simulink model "Kugle_sys7_block"  (R2018b)
settings: Solver=VariableStepAuto  StartTime=0.0  StopTime=10.0  RelTol=1e-3
settings Model: Creator=martinandersen  LastModifiedBy=martinandersen

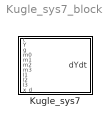
== system Kugle_sys7_block ==
  Kugle_sys7 : MATLAB Function  TreatAsAtomicUnit=on

== matlab function Kugle_sys7_block/Kugle_sys7 ==
  data: t input; dYdt output; Y input; g input; m0 input; m1 input; m2 input; m3 input; l1 input; l2 input; l3 input; x_d input
function dYdt = Kugle_sys7(t,Y,g,m0,m1,m2,m3,l1,l2,l3,x_d)
%#codegen

%    This function was generated by the Symbolic Math Toolbox version 8.2.
%    11-May-2019 12:19:22

t3 = Y(3);
t2 = cos(t3);
t4 = t2.^2;
t5 = m3.^2;
t7 = Y(5);
t6 = cos(t7);
t11 = t3+t7;
t8 = cos(t11);
t9 = m2.^2;
t10 = t6.^2;
t12 = t8.^2;
t13 = Y(1);
t14 = sin(t13);
t15 = Y(2);
t16 = sin(t3);
t17 = t15.^2;
t18 = Y(4);
t19 = t18.^2;
t20 = t3+t13;
t21 = sin(t20);
t22 = sin(t11);
t23 = Y(6);
t24 = t23.^2;
t25 = sin(t7);
t26 = t3+t7+t13;
t27 = sin(t26);
t28 = 1.0./l1;
t29 = t4.*t9.*9.0;
t30 = t4.*t5.*3.6e1;
t31 = t5.*t10.*2.7e1;
t32 = t5.*t12.*2.7e1;
t33 = m2.*m3.*t4.*3.6e1;
t34 = m1.*m3.*t10.*9.0;
t35 = m2.*m3.*t10.*2.7e1;
t36 = m2.*m3.*t12.*9.0;
t37 = t5.*-3.6e1-t9.*1.2e1+t29+t30+t31+t32+t33+t34+t35+t36-m1.*m2.*4.0-m1.*m3.*1.2e1-m2.*m3.*4.8e1-t2.*t5.*t6.*t8.*5.4e1-m2.*m3.*t2.*t6.*t8.*2.7e1;
t38 = 1.0./t37;
t39 = l1.^2;
t40 = l2.^2;
t41 = l3.^2;
dYdt = [t15;t28.*t38.*(g.*t5.*t14.*2.4e1+g.*t9.*t14.*8.0+g.*m1.*m2.*t14.*4.0+g.*m1.*m3.*t14.*1.2e1+g.*m2.*m3.*t14.*3.2e1-g.*t2.*t5.*t21.*2.4e1-g.*t5.*t10.*t14.*1.8e1-g.*t2.*t9.*t21.*6.0-g.*t5.*t8.*t27.*1.8e1+l2.*t5.*t16.*t17.*2.4e1+l2.*t5.*t16.*t19.*2.4e1+l2.*t9.*t16.*t17.*4.0+l2.*t9.*t16.*t19.*4.0+l3.*t5.*t17.*t22.*1.2e1+l3.*t5.*t19.*t22.*1.2e1+l3.*t5.*t22.*t24.*1.2e1-g.*m1.*m3.*t10.*t14.*9.0-g.*m2.*m3.*t2.*t21.*2.4e1-g.*m2.*m3.*t10.*t14.*1.8e1-g.*m2.*m3.*t8.*t27.*6.0+l2.*m2.*m3.*t16.*t17.*2.0e1+l2.*m2.*m3.*t16.*t19.*2.0e1+l3.*m2.*m3.*t17.*t22.*4.0+l3.*m2.*m3.*t19.*t22.*4.0+l3.*m2.*m3.*t22.*t24.*4.0+g.*t2.*t5.*t6.*t27.*1.8e1+g.*t5.*t6.*t8.*t21.*1.8e1+l1.*t2.*t5.*t16.*t17.*2.4e1+l1.*t2.*t9.*t16.*t17.*6.0-l2.*t5.*t10.*t16.*t17.*1.8e1-l2.*t5.*t10.*t16.*t19.*1.8e1-l3.*t2.*t5.*t17.*t25.*1.2e1+l1.*t5.*t8.*t17.*t22.*1.8e1-l3.*t2.*t5.*t19.*t25.*1.2e1+l2.*t5.*t15.*t16.*t18.*4.8e1+l2.*t5.*t8.*t17.*t25.*1.8e1-l3.*t5.*t10.*t17.*t22.*9.0+l2.*t5.*t8.*t19.*t25.*1.8e1-l3.*t2.*t5.*t24.*t25.*1.2e1-l3.*t5.*t10.*t19.*t22.*9.0+l2.*t9.*t15.*t16.*t18.*8.0+l3.*t5.*t15.*t18.*t22.*2.4e1-l3.*t5.*t10.*t22.*t24.*9.0+l3.*t5.*t15.*t22.*t23.*2.4e1+l3.*t5.*t18.*t22.*t23.*2.4e1+l1.*m2.*m3.*t2.*t16.*t17.*2.4e1-l2.*m2.*m3.*t10.*t16.*t17.*9.0-l2.*m2.*m3.*t10.*t16.*t19.*9.0-l3.*m2.*m3.*t2.*t17.*t25.*6.0+l1.*m2.*m3.*t8.*t17.*t22.*6.0-l3.*m2.*m3.*t2.*t19.*t25.*6.0+l2.*m2.*m3.*t15.*t16.*t18.*4.0e1+l2.*m2.*m3.*t8.*t17.*t25.*6.0+l2.*m2.*m3.*t8.*t19.*t25.*6.0-l3.*m2.*m3.*t2.*t24.*t25.*6.0+l3.*m2.*m3.*t15.*t18.*t22.*8.0+l3.*m2.*m3.*t15.*t22.*t23.*8.0+l3.*m2.*m3.*t18.*t22.*t23.*8.0-l1.*t2.*t5.*t6.*t17.*t22.*1.8e1-l1.*t5.*t6.*t8.*t16.*t17.*1.8e1-l2.*t2.*t5.*t6.*t17.*t25.*1.8e1-l2.*t2.*t5.*t6.*t19.*t25.*1.8e1+l3.*t5.*t6.*t8.*t17.*t25.*9.0-l2.*t5.*t10.*t15.*t16.*t18.*3.6e1+l3.*t5.*t6.*t8.*t19.*t25.*9.0-l3.*t2.*t5.*t15.*t18.*t25.*2.4e1+l3.*t5.*t6.*t8.*t24.*t25.*9.0+l2.*t5.*t8.*t15.*t18.*t25.*3.6e1-l3.*t2.*t5.*t15.*t23.*t25.*2.4e1-l3.*t5.*t10.*t15.*t18.*t22.*1.8e1-l3.*t2.*t5.*t18.*t23.*t25.*2.4e1-l3.*t5.*t10.*t15.*t22.*t23.*1.8e1-l3.*t5.*t10.*t18.*t22.*t23.*1.8e1+g.*m2.*m3.*t2.*t6.*t27.*9.0+g.*m2.*m3.*t6.*t8.*t21.*9.0-l1.*m2.*m3.*t2.*t6.*t17.*t22.*9.0-l1.*m2.*m3.*t6.*t8.*t16.*t17.*9.0-l2.*m2.*m3.*t2.*t6.*t17.*t25.*9.0-l2.*m2.*m3.*t2.*t6.*t19.*t25.*9.0-l2.*m2.*m3.*t10.*t15.*t16.*t18.*1.8e1-l3.*m2.*m3.*t2.*t15.*t18.*t25.*1.2e1+l2.*m2.*m3.*t8.*t15.*t18.*t25.*1.2e1-l3.*m2.*m3.*t2.*t15.*t23.*t25.*1.2e1-l3.*m2.*m3.*t2.*t18.*t23.*t25.*1.2e1-l2.*t2.*t5.*t6.*t15.*t18.*t25.*3.6e1+l3.*t5.*t6.*t8.*t15.*t18.*t25.*1.8e1+l3.*t5.*t6.*t8.*t15.*t23.*t25.*1.8e1+l3.*t5.*t6.*t8.*t18.*t23.*t25.*1.8e1-l2.*m2.*m3.*t2.*t6.*t15.*t18.*t25.*1.8e1).*(-3.0./2.0);t18;(t28.*t38.*(g.*l2.*t5.*t14.*2.4e1+g.*l2.*t9.*t14.*8.0-g.*l1.*t5.*t21.*2.4e1-g.*l1.*t9.*t21.*1.2e1+t5.*t16.*t17.*t39.*2.4e1+t5.*t16.*t17.*t40.*2.4e1+t5.*t16.*t19.*t40.*2.4e1+t9.*t16.*t17.*t39.*1.2e1+t9.*t16.*t17.*t40.*4.0+t9.*t16.*t19.*t40.*4.0+g.*l2.*m1.*m2.*t14.*4.0+g.*l2.*m1.*m3.*t14.*1.2e1+g.*l2.*m2.*m3.*t14.*3.2e1-g.*l1.*m1.*m2.*t21.*4.0-g.*l1.*m1.*m3.*t21.*8.0-g.*l1.*m2.*m3.*t21.*3.6e1+g.*l1.*t2.*t5.*t14.*2.4e1+g.*l1.*t2.*t9.*t14.*1.2e1-g.*l2.*t2.*t5.*t21.*2.4e1-g.*l2.*t5.*t10.*t14.*1.8e1-g.*l2.*t2.*t9.*t21.*6.0+g.*l1.*t5.*t6.*t27.*1.8e1+g.*l1.*t5.*t12.*t21.*1.8e1-g.*l2.*t5.*t8.*t27.*1.8e1+l2.*l3.*t5.*t17.*t22.*1.2e1-l1.*l3.*t5.*t17.*t25.*1.2e1+l2.*l3.*t5.*t19.*t22.*1.2e1-l1.*l3.*t5.*t19.*t25.*1.2e1+l2.*l3.*t5.*t22.*t24.*1.2e1-l1.*l3.*t5.*t24.*t25.*1.2e1+m1.*m2.*t16.*t17.*t39.*4.0+m1.*m3.*t16.*t17.*t39.*8.0+m2.*m3.*t16.*t17.*t39.*3.6e1+m2.*m3.*t16.*t17.*t40.*2.0e1+m2.*m3.*t16.*t19.*t40.*2.0e1-t5.*t10.*t16.*t17.*t40.*1.8e1-t5.*t6.*t17.*t22.*t39.*1.8e1-t5.*t12.*t16.*t17.*t39.*1.8e1-t5.*t10.*t16.*t19.*t40.*1.8e1+t5.*t15.*t16.*t18.*t40.*4.8e1+t5.*t8.*t17.*t25.*t40.*1.8e1+t5.*t8.*t19.*t25.*t40.*1.8e1+t9.*t15.*t16.*t18.*t40.*8.0-g.*l1.*t5.*t6.*t8.*t14.*1.8e1+g.*l2.*t2.*t5.*t6.*t27.*1.8e1+g.*l2.*t5.*t6.*t8.*t21.*1.8e1-g.*l1.*t2.*t5.*t8.*t27.*1.8e1+l1.*l2.*t2.*t5.*t16.*t17.*4.8e1+l1.*l2.*t2.*t5.*t16.*t19.*2.4e1+l1.*l2.*t2.*t9.*t16.*t17.*1.2e1+l1.*l2.*t2.*t9.*t16.*t19.*6.0+l1.*l3.*t2.*t5.*t17.*t22.*1.2e1+l1.*l3.*t2.*t5.*t19.*t22.*1.2e1-l2.*l3.*t2.*t5.*t17.*t25.*1.2e1+l1.*l2.*t5.*t8.*t17.*t22.*1.8e1-l1.*l2.*t5.*t6.*t17.*t25.*1.8e1-l2.*l3.*t2.*t5.*t19.*t25.*1.2e1+l1.*l3.*t2.*t5.*t22.*t24.*1.2e1-l1.*l2.*t5.*t6.*t19.*t25.*1.8e1-l2.*l3.*t5.*t10.*t17.*t22.*9.0-l2.*l3.*t2.*t5.*t24.*t25.*1.2e1-l2.*l3.*t5.*t10.*t19.*t22.*9.0+l1.*l3.*t5.*t12.*t17.*t25.*9.0+l1.*l3.*t5.*t12.*t19.*t25.*9.0+l2.*l3.*t5.*t15.*t18.*t22.*2.4e1-l2.*l3.*t5.*t10.*t22.*t24.*9.0-l1.*l3.*t5.*t15.*t18.*t25.*2.4e1+l1.*l3.*t5.*t12.*t24.*t25.*9.0+l2.*l3.*t5.*t15.*t22.*t23.*2.4e1-l1.*l3.*t5.*t15.*t23.*t25.*2.4e1+l2.*l3.*t5.*t18.*t22.*t23.*2.4e1-l1.*l3.*t5.*t18.*t23.*t25.*2.4e1-m1.*m3.*t6.*t17.*t22.*t39.*6.0-m2.*m3.*t10.*t16.*t17.*t40.*9.0-m2.*m3.*t6.*t17.*t22.*t39.*1.8e1-m2.*m3.*t12.*t16.*t17.*t39.*9.0-m2.*m3.*t10.*t16.*t19.*t40.*9.0+m2.*m3.*t15.*t16.*t18.*t40.*4.0e1+m2.*m3.*t8.*t17.*t25.*t40.*6.0+m2.*m3.*t8.*t19.*t25.*t40.*6.0+t2.*t5.*t8.*t17.*t22.*t39.*1.8e1-t2.*t5.*t6.*t17.*t25.*t40.*1.8e1-t2.*t5.*t6.*t19.*t25.*t40.*1.8e1-t5.*t10.*t15.*t16.*t18.*t40.*3.6e1+t5.*t8.*t15.*t18.*t25.*t40.*3.6e1+g.*l1.*m1.*m2.*t2.*t14.*6.0+g.*l1.*m1.*m3.*t2.*t14.*1.2e1+g.*l1.*m2.*m3.*t2.*t14.*3.6e1-g.*l2.*m1.*m3.*t10.*t14.*9.0-g.*l2.*m2.*m3.*t2.*t21.*2.4e1-g.*l2.*m2.*m3.*t10.*t14.*1.8e1+g.*l1.*m1.*m3.*t6.*t27.*6.0+g.*l1.*m2.*m3.*t6.*t27.*1.8e1+g.*l1.*m2.*m3.*t12.*t21.*9.0-g.*l2.*m2.*m3.*t8.*t27.*6.0+l2.*l3.*m2.*m3.*t17.*t22.*4.0-l1.*l3.*m1.*m3.*t17.*t25.*4.0-l1.*l3.*m2.*m3.*t17.*t25.*1.2e1+l2.*l3.*m2.*m3.*t19.*t22.*4.0-l1.*l3.*m1.*m3.*t19.*t25.*4.0-l1.*l3.*m2.*m3.*t19.*t25.*1.2e1+l2.*l3.*m2.*m3.*t22.*t24.*4.0-l1.*l3.*m1.*m3.*t24.*t25.*4.0-l1.*l3.*m2.*m3.*t24.*t25.*1.2e1-g.*l1.*m1.*m3.*t6.*t8.*t14.*9.0-g.*l1.*m2.*m3.*t6.*t8.*t14.*1.8e1+g.*l2.*m2.*m3.*t2.*t6.*t27.*9.0+g.*l2.*m2.*m3.*t6.*t8.*t21.*9.0-g.*l1.*m2.*m3.*t2.*t8.*t27.*9.0+l1.*l2.*m2.*m3.*t2.*t16.*t17.*4.8e1+l1.*l2.*m2.*m3.*t2.*t16.*t19.*2.4e1+l1.*l3.*m2.*m3.*t2.*t17.*t22.*6.0+l1.*l3.*m2.*m3.*t2.*t19.*t22.*6.0-l2.*l3.*m2.*m3.*t2.*t17.*t25.*6.0-l1.*l2.*m1.*m3.*t6.*t17.*t25.*6.0+l1.*l2.*m2.*m3.*t8.*t17.*t22.*6.0-l1.*l2.*m2.*m3.*t6.*t17.*t25.*1.8e1-l2.*l3.*m2.*m3.*t2.*t19.*t25.*6.0-l1.*l2.*m1.*m3.*t6.*t19.*t25.*6.0+l1.*l3.*m2.*m3.*t2.*t22.*t24.*6.0-l1.*l2.*m2.*m3.*t6.*t19.*t25.*1.8e1-l2.*l3.*m2.*m3.*t2.*t24.*t25.*6.0+l2.*l3.*m2.*m3.*t15.*t18.*t22.*8.0-l1.*l3.*m1.*m3.*t15.*t18.*t25.*8.0-l1.*l3.*m2.*m3.*t15.*t18.*t25.*2.4e1+l2.*l3.*m2.*m3.*t15.*t22.*t23.*8.0-l1.*l3.*m1.*m3.*t15.*t23.*t25.*8.0-l1.*l3.*m2.*m3.*t15.*t23.*t25.*2.4e1+l2.*l3.*m2.*m3.*t18.*t22.*t23.*8.0-l1.*l3.*m1.*m3.*t18.*t23.*t25.*8.0-l1.*l3.*m2.*m3.*t18.*t23.*t25.*2.4e1-l1.*l2.*t2.*t5.*t6.*t17.*t22.*1.8e1-l1.*l2.*t5.*t6.*t8.*t16.*t17.*3.6e1-l1.*l2.*t5.*t6.*t8.*t16.*t19.*1.8e1+l1.*l2.*t2.*t5.*t15.*t16.*t18.*4.8e1+l1.*l2.*t2.*t5.*t8.*t17.*t25.*1.8e1+l1.*l2.*t2.*t5.*t8.*t19.*t25.*1.8e1-l1.*l3.*t5.*t6.*t8.*t17.*t22.*9.0+l1.*l2.*t2.*t9.*t15.*t16.*t18.*1.2e1-l1.*l3.*t5.*t6.*t8.*t19.*t22.*9.0+l1.*l3.*t2.*t5.*t15.*t18.*t22.*2.4e1+l2.*l3.*t5.*t6.*t8.*t17.*t25.*9.0+l2.*l3.*t5.*t6.*t8.*t19.*t25.*9.0-l1.*l3.*t5.*t6.*t8.*t22.*t24.*9.0-l2.*l3.*t2.*t5.*t15.*t18.*t25.*2.4e1+l1.*l3.*t2.*t5.*t15.*t22.*t23.*2.4e1-l1.*l2.*t5.*t6.*t15.*t18.*t25.*3.6e1+l2.*l3.*t5.*t6.*t8.*t24.*t25.*9.0+l1.*l3.*t2.*t5.*t18.*t22.*t23.*2.4e1-l2.*l3.*t2.*t5.*t15.*t23.*t25.*2.4e1-l2.*l3.*t5.*t10.*t15.*t18.*t22.*1.8e1-l2.*l3.*t2.*t5.*t18.*t23.*t25.*2.4e1+l1.*l3.*t5.*t12.*t15.*t18.*t25.*1.8e1-l2.*l3.*t5.*t10.*t15.*t22.*t23.*1.8e1-l2.*l3.*t5.*t10.*t18.*t22.*t23.*1.8e1+l1.*l3.*t5.*t12.*t15.*t23.*t25.*1.8e1+l1.*l3.*t5.*t12.*t18.*t23.*t25.*1.8e1+m2.*m3.*t2.*t8.*t17.*t22.*t39.*9.0-m2.*m3.*t2.*t6.*t17.*t25.*t40.*9.0-m2.*m3.*t2.*t6.*t19.*t25.*t40.*9.0-m2.*m3.*t10.*t15.*t16.*t18.*t40.*1.8e1+m2.*m3.*t8.*t15.*t18.*t25.*t40.*1.2e1-t2.*t5.*t6.*t15.*t18.*t25.*t40.*3.6e1-l1.*l2.*m2.*m3.*t2.*t6.*t17.*t22.*9.0-l1.*l2.*m2.*m3.*t6.*t8.*t16.*t17.*1.8e1-l1.*l2.*m2.*m3.*t6.*t8.*t16.*t19.*9.0+l1.*l2.*m2.*m3.*t2.*t15.*t16.*t18.*4.8e1+l1.*l2.*m2.*m3.*t2.*t8.*t17.*t25.*9.0+l1.*l2.*m2.*m3.*t2.*t8.*t19.*t25.*9.0+l1.*l3.*m2.*m3.*t2.*t15.*t18.*t22.*1.2e1-l2.*l3.*m2.*m3.*t2.*t15.*t18.*t25.*1.2e1-l1.*l2.*m1.*m3.*t6.*t15.*t18.*t25.*1.2e1+l1.*l3.*m2.*m3.*t2.*t15.*t22.*t23.*1.2e1-l1.*l2.*m2.*m3.*t6.*t15.*t18.*t25.*3.6e1+l1.*l3.*m2.*m3.*t2.*t18.*t22.*t23.*1.2e1-l2.*l3.*m2.*m3.*t2.*t15.*t23.*t25.*1.2e1-l2.*l3.*m2.*m3.*t2.*t18.*t23.*t25.*1.2e1-l1.*l2.*t5.*t6.*t8.*t15.*t16.*t18.*3.6e1+l1.*l2.*t2.*t5.*t8.*t15.*t18.*t25.*3.6e1-l1.*l3.*t5.*t6.*t8.*t15.*t18.*t22.*1.8e1+l2.*l3.*t5.*t6.*t8.*t15.*t18.*t25.*1.8e1-l1.*l3.*t5.*t6.*t8.*t15.*t22.*t23.*1.8e1-l1.*l3.*t5.*t6.*t8.*t18.*t22.*t23.*1.8e1+l2.*l3.*t5.*t6.*t8.*t15.*t23.*t25.*1.8e1+l2.*l3.*t5.*t6.*t8.*t18.*t23.*t25.*1.8e1-m2.*m3.*t2.*t6.*t15.*t18.*t25.*t40.*1.8e1-l1.*l2.*m2.*m3.*t6.*t8.*t15.*t16.*t18.*1.8e1+l1.*l2.*m2.*m3.*t2.*t8.*t15.*t18.*t25.*1.8e1).*(3.0./2.0))./l2;t23;((g.*l3.*t5.*t21.*2.4e1+g.*l3.*t9.*t21.*1.2e1-g.*l2.*t5.*t27.*3.6e1-g.*l2.*t9.*t27.*1.2e1+t5.*t17.*t25.*t40.*3.6e1+t5.*t17.*t25.*t41.*1.2e1+t5.*t19.*t25.*t40.*3.6e1+t5.*t19.*t25.*t41.*1.2e1+t9.*t17.*t25.*t40.*1.2e1+t9.*t19.*t25.*t40.*1.2e1+t5.*t24.*t25.*t41.*1.2e1+g.*l3.*m1.*m2.*t21.*4.0+g.*l3.*m1.*m3.*t21.*8.0+g.*l3.*m2.*m3.*t21.*3.6e1-g.*l2.*m1.*m2.*t27.*4.0-g.*l2.*m1.*m3.*t27.*1.2e1-g.*l2.*m2.*m3.*t27.*4.8e1-g.*l3.*t2.*t5.*t14.*2.4e1-g.*l3.*t2.*t9.*t14.*1.2e1+g.*l2.*t5.*t8.*t14.*3.6e1+g.*l2.*t8.*t9.*t14.*1.2e1+g.*l2.*t5.*t6.*t21.*3.6e1+g.*l2.*t4.*t5.*t27.*3.6e1+g.*l2.*t6.*t9.*t21.*1.8e1-g.*l3.*t5.*t6.*t27.*1.8e1-g.*l3.*t5.*t12.*t21.*1.8e1+g.*l2.*t4.*t9.*t27.*9.0-l1.*l3.*t5.*t16.*t17.*2.4e1-l1.*l3.*t9.*t16.*t17.*1.2e1+l1.*l2.*t5.*t17.*t22.*3.6e1+l1.*l2.*t9.*t17.*t22.*1.2e1+m1.*m2.*t17.*t25.*t40.*4.0+m1.*m3.*t17.*t25.*t40.*1.2e1+m1.*m2.*t19.*t25.*t40.*4.0+m1.*m3.*t17.*t25.*t41.*4.0+m2.*m3.*t17.*t25.*t40.*4.8e1+m1.*m3.*t19.*t25.*t40.*1.2e1+m2.*m3.*t17.*t25.*t41.*1.2e1+m1.*m3.*t19.*t25.*t41.*4.0+m2.*m3.*t19.*t25.*t40.*4.8e1+m2.*m3.*t19.*t25.*t41.*1.2e1+m1.*m3.*t24.*t25.*t41.*4.0+m2.*m3.*t24.*t25.*t41.*1.2e1+t5.*t8.*t16.*t17.*t40.*3.6e1-t2.*t5.*t17.*t22.*t41.*1.2e1+t5.*t8.*t16.*t19.*t40.*3.6e1-t2.*t5.*t19.*t22.*t41.*1.2e1+t8.*t9.*t16.*t17.*t40.*6.0-t4.*t5.*t17.*t25.*t40.*3.6e1+t8.*t9.*t16.*t19.*t40.*6.0-t4.*t5.*t19.*t25.*t40.*3.6e1-t2.*t5.*t22.*t24.*t41.*1.2e1-t4.*t9.*t17.*t25.*t40.*9.0-t4.*t9.*t19.*t25.*t40.*9.0-t5.*t12.*t17.*t25.*t41.*9.0-t5.*t12.*t19.*t25.*t41.*9.0+t5.*t15.*t18.*t25.*t40.*7.2e1+t5.*t15.*t18.*t25.*t41.*2.4e1-t5.*t12.*t24.*t25.*t41.*9.0+t9.*t15.*t18.*t25.*t40.*2.4e1+t5.*t15.*t23.*t25.*t41.*2.4e1+t5.*t18.*t23.*t25.*t41.*2.4e1-g.*l2.*t2.*t5.*t6.*t14.*3.6e1-g.*l2.*t2.*t6.*t9.*t14.*1.8e1+g.*l3.*t5.*t6.*t8.*t14.*1.8e1-g.*l2.*t2.*t5.*t8.*t21.*3.6e1-g.*l2.*t2.*t8.*t9.*t21.*9.0+g.*l3.*t2.*t5.*t8.*t27.*1.8e1-l2.*l3.*t2.*t5.*t16.*t17.*2.4e1-l1.*l2.*t5.*t6.*t16.*t17.*3.6e1-l2.*l3.*t2.*t5.*t16.*t19.*2.4e1-l2.*l3.*t2.*t9.*t16.*t17.*6.0-l1.*l2.*t4.*t5.*t17.*t22.*3.6e1-l1.*l2.*t6.*t9.*t16.*t17.*1.8e1-l2.*l3.*t2.*t9.*t16.*t19.*6.0+l1.*l3.*t5.*t6.*t17.*t22.*1.8e1+l1.*l3.*t5.*t12.*t16.*t17.*1.8e1-l1.*l2.*t4.*t9.*t17.*t22.*9.0+l2.*l3.*t5.*t8.*t17.*t22.*1.8e1+l2.*l3.*t5.*t6.*t17.*t25.*3.6e1+l2.*l3.*t5.*t8.*t19.*t22.*1.8e1+l2.*l3.*t5.*t6.*t19.*t25.*3.6e1+l2.*l3.*t5.*t8.*t22.*t24.*1.8e1+l2.*l3.*t5.*t6.*t24.*t25.*1.8e1+m2.*m3.*t8.*t16.*t17.*t40.*3.0e1-m2.*m3.*t2.*t17.*t22.*t41.*6.0+m2.*m3.*t8.*t16.*t19.*t40.*3.0e1-m2.*m3.*t2.*t19.*t22.*t41.*6.0-m2.*m3.*t4.*t17.*t25.*t40.*3.6e1-m2.*m3.*t4.*t19.*t25.*t40.*3.6e1-m2.*m3.*t2.*t22.*t24.*t41.*6.0+m1.*m2.*t15.*t18.*t25.*t40.*8.0+m1.*m3.*t15.*t18.*t25.*t40.*2.4e1+m1.*m3.*t15.*t18.*t25.*t41.*8.0+m2.*m3.*t15.*t18.*t25.*t40.*9.6e1+m2.*m3.*t15.*t18.*t25.*t41.*2.4e1+m1.*m3.*t15.*t23.*t25.*t41.*8.0+m2.*m3.*t15.*t23.*t25.*t41.*2.4e1+m1.*m3.*t18.*t23.*t25.*t41.*8.0+m2.*m3.*t18.*t23.*t25.*t41.*2.4e1-t2.*t5.*t6.*t16.*t17.*t40.*3.6e1-t2.*t5.*t6.*t16.*t19.*t40.*3.6e1-t2.*t6.*t9.*t16.*t17.*t40.*9.0-t2.*t6.*t9.*t16.*t19.*t40.*9.0+t5.*t6.*t8.*t17.*t22.*t41.*9.0+t5.*t6.*t8.*t19.*t22.*t41.*9.0+t5.*t8.*t15.*t16.*t18.*t40.*7.2e1-t2.*t5.*t15.*t18.*t22.*t41.*2.4e1+t5.*t6.*t8.*t22.*t24.*t41.*9.0+t8.*t9.*t15.*t16.*t18.*t40.*1.2e1-t4.*t5.*t15.*t18.*t25.*t40.*7.2e1-t2.*t5.*t15.*t22.*t23.*t41.*2.4e1-t2.*t5.*t18.*t22.*t23.*t41.*2.4e1-t4.*t9.*t15.*t18.*t25.*t40.*1.8e1-t5.*t12.*t15.*t18.*t25.*t41.*1.8e1-t5.*t12.*t15.*t23.*t25.*t41.*1.8e1-t5.*t12.*t18.*t23.*t25.*t41.*1.8e1-g.*l3.*m1.*m2.*t2.*t14.*6.0-g.*l3.*m1.*m3.*t2.*t14.*1.2e1-g.*l3.*m2.*m3.*t2.*t14.*3.6e1+g.*l2.*m1.*m2.*t8.*t14.*6.0+g.*l2.*m1.*m3.*t8.*t14.*1.8e1+g.*l2.*m2.*m3.*t8.*t14.*4.8e1+g.*l2.*m1.*m2.*t6.*t21.*6.0+g.*l2.*m1.*m3.*t6.*t21.*1.2e1+g.*l2.*m2.*m3.*t6.*t21.*5.4e1+g.*l2.*m2.*m3.*t4.*t27.*3.6e1-g.*l3.*m1.*m3.*t6.*t27.*6.0-g.*l3.*m2.*m3.*t6.*t27.*1.8e1-g.*l3.*m2.*m3.*t12.*t21.*9.0-l1.*l3.*m1.*m2.*t16.*t17.*4.0-l1.*l3.*m1.*m3.*t16.*t17.*8.0-l1.*l3.*m2.*m3.*t16.*t17.*3.6e1+l1.*l2.*m1.*m2.*t17.*t22.*4.0+l1.*l2.*m1.*m3.*t17.*t22.*1.2e1+l1.*l2.*m2.*m3.*t17.*t22.*4.8e1-g.*l2.*m1.*m2.*t2.*t6.*t14.*9.0-g.*l2.*m1.*m3.*t2.*t6.*t14.*1.8e1-g.*l2.*m2.*m3.*t2.*t6.*t14.*5.4e1+g.*l3.*m1.*m3.*t6.*t8.*t14.*9.0+g.*l3.*m2.*m3.*t6.*t8.*t14.*1.8e1-g.*l2.*m2.*m3.*t2.*t8.*t21.*3.6e1+g.*l3.*m2.*m3.*t2.*t8.*t27.*9.0-l1.*l2.*m1.*m2.*t6.*t16.*t17.*6.0-l2.*l3.*m2.*m3.*t2.*t16.*t17.*2.4e1-l1.*l2.*m1.*m3.*t6.*t16.*t17.*1.2e1-l1.*l2.*m2.*m3.*t6.*t16.*t17.*5.4e1-l2.*l3.*m2.*m3.*t2.*t16.*t19.*2.4e1-l1.*l2.*m2.*m3.*t4.*t17.*t22.*3.6e1+l1.*l3.*m1.*m3.*t6.*t17.*t22.*6.0+l1.*l3.*m2.*m3.*t6.*t17.*t22.*1.8e1+l1.*l3.*m2.*m3.*t12.*t16.*t17.*9.0+l2.*l3.*m1.*m3.*t6.*t17.*t25.*1.2e1+l2.*l3.*m2.*m3.*t8.*t17.*t22.*6.0+l2.*l3.*m2.*m3.*t6.*t17.*t25.*3.6e1+l2.*l3.*m1.*m3.*t6.*t19.*t25.*1.2e1+l2.*l3.*m2.*m3.*t8.*t19.*t22.*6.0+l2.*l3.*m2.*m3.*t6.*t19.*t25.*3.6e1+l2.*l3.*m1.*m3.*t6.*t24.*t25.*6.0+l2.*l3.*m2.*m3.*t8.*t22.*t24.*6.0+l2.*l3.*m2.*m3.*t6.*t24.*t25.*1.8e1+l1.*l2.*t2.*t5.*t8.*t16.*t17.*3.6e1+l1.*l2.*t2.*t8.*t9.*t16.*t17.*9.0-l2.*l3.*t2.*t5.*t6.*t17.*t22.*1.8e1+l2.*l3.*t5.*t6.*t8.*t16.*t17.*1.8e1-l1.*l3.*t2.*t5.*t8.*t17.*t22.*1.8e1-l2.*l3.*t2.*t5.*t6.*t19.*t22.*1.8e1+l2.*l3.*t5.*t6.*t8.*t16.*t19.*1.8e1-l2.*l3.*t2.*t5.*t15.*t16.*t18.*4.8e1-l2.*l3.*t2.*t5.*t8.*t17.*t25.*3.6e1-l2.*l3.*t2.*t5.*t6.*t22.*t24.*1.8e1-l2.*l3.*t2.*t5.*t8.*t19.*t25.*3.6e1-l2.*l3.*t2.*t9.*t15.*t16.*t18.*1.2e1-l2.*l3.*t2.*t5.*t8.*t24.*t25.*1.8e1+l2.*l3.*t5.*t8.*t15.*t18.*t22.*3.6e1+l2.*l3.*t5.*t6.*t15.*t18.*t25.*7.2e1+l2.*l3.*t5.*t8.*t15.*t22.*t23.*3.6e1+l2.*l3.*t5.*t6.*t15.*t23.*t25.*3.6e1+l2.*l3.*t5.*t8.*t18.*t22.*t23.*3.6e1+l2.*l3.*t5.*t6.*t18.*t23.*t25.*3.6e1-m2.*m3.*t2.*t6.*t16.*t17.*t40.*3.6e1-m2.*m3.*t2.*t6.*t16.*t19.*t40.*3.6e1+m2.*m3.*t8.*t15.*t16.*t18.*t40.*6.0e1-m2.*m3.*t2.*t15.*t18.*t22.*t41.*1.2e1-m2.*m3.*t4.*t15.*t18.*t25.*t40.*7.2e1-m2.*m3.*t2.*t15.*t22.*t23.*t41.*1.2e1-m2.*m3.*t2.*t18.*t22.*t23.*t41.*1.2e1-t2.*t5.*t6.*t15.*t16.*t18.*t40.*7.2e1-t2.*t6.*t9.*t15.*t16.*t18.*t40.*1.8e1+t5.*t6.*t8.*t15.*t18.*t22.*t41.*1.8e1+t5.*t6.*t8.*t15.*t22.*t23.*t41.*1.8e1+t5.*t6.*t8.*t18.*t22.*t23.*t41.*1.8e1+l1.*l2.*m2.*m3.*t2.*t8.*t16.*t17.*3.6e1-l2.*l3.*m2.*m3.*t2.*t6.*t17.*t22.*9.0+l2.*l3.*m2.*m3.*t6.*t8.*t16.*t17.*9.0-l1.*l3.*m2.*m3.*t2.*t8.*t17.*t22.*9.0-l2.*l3.*m2.*m3.*t2.*t6.*t19.*t22.*9.0+l2.*l3.*m2.*m3.*t6.*t8.*t16.*t19.*9.0-l2.*l3.*m2.*m3.*t2.*t15.*t16.*t18.*4.8e1-l2.*l3.*m2.*m3.*t2.*t8.*t17.*t25.*1.8e1-l2.*l3.*m2.*m3.*t2.*t6.*t22.*t24.*9.0-l2.*l3.*m2.*m3.*t2.*t8.*t19.*t25.*1.8e1-l2.*l3.*m2.*m3.*t2.*t8.*t24.*t25.*9.0+l2.*l3.*m1.*m3.*t6.*t15.*t18.*t25.*2.4e1+l2.*l3.*m2.*m3.*t8.*t15.*t18.*t22.*1.2e1+l2.*l3.*m2.*m3.*t6.*t15.*t18.*t25.*7.2e1+l2.*l3.*m1.*m3.*t6.*t15.*t23.*t25.*1.2e1+l2.*l3.*m2.*m3.*t8.*t15.*t22.*t23.*1.2e1+l2.*l3.*m2.*m3.*t6.*t15.*t23.*t25.*3.6e1+l2.*l3.*m1.*m3.*t6.*t18.*t23.*t25.*1.2e1+l2.*l3.*m2.*m3.*t8.*t18.*t22.*t23.*1.2e1+l2.*l3.*m2.*m3.*t6.*t18.*t23.*t25.*3.6e1-l2.*l3.*t2.*t5.*t6.*t15.*t18.*t22.*3.6e1+l2.*l3.*t5.*t6.*t8.*t15.*t16.*t18.*3.6e1-l2.*l3.*t2.*t5.*t6.*t15.*t22.*t23.*3.6e1-l2.*l3.*t2.*t5.*t8.*t15.*t18.*t25.*7.2e1-l2.*l3.*t2.*t5.*t6.*t18.*t22.*t23.*3.6e1-l2.*l3.*t2.*t5.*t8.*t15.*t23.*t25.*3.6e1-l2.*l3.*t2.*t5.*t8.*t18.*t23.*t25.*3.6e1-m2.*m3.*t2.*t6.*t15.*t16.*t18.*t40.*7.2e1-l2.*l3.*m2.*m3.*t2.*t6.*t15.*t18.*t22.*1.8e1+l2.*l3.*m2.*m3.*t6.*t8.*t15.*t16.*t18.*1.8e1-l2.*l3.*m2.*m3.*t2.*t6.*t15.*t22.*t23.*1.8e1-l2.*l3.*m2.*m3.*t2.*t8.*t15.*t18.*t25.*3.6e1-l2.*l3.*m2.*m3.*t2.*t6.*t18.*t22.*t23.*1.8e1-l2.*l3.*m2.*m3.*t2.*t8.*t15.*t23.*t25.*1.8e1-l2.*l3.*m2.*m3.*t2.*t8.*t18.*t23.*t25.*1.8e1).*(3.0./2.0))./(l2.*l3.*t5.*-3.6e1-l2.*l3.*t9.*1.2e1-l2.*l3.*m1.*m2.*4.0-l2.*l3.*m1.*m3.*1.2e1-l2.*l3.*m2.*m3.*4.8e1+l2.*l3.*t4.*t5.*3.6e1+l2.*l3.*t4.*t9.*9.0+l2.*l3.*t5.*t10.*2.7e1+l2.*l3.*t5.*t12.*2.7e1+l2.*l3.*m2.*m3.*t4.*3.6e1+l2.*l3.*m1.*m3.*t10.*9.0+l2.*l3.*m2.*m3.*t10.*2.7e1+l2.*l3.*m2.*m3.*t12.*9.0-l2.*l3.*t2.*t5.*t6.*t8.*5.4e1-l2.*l3.*m2.*m3.*t2.*t6.*t8.*2.7e1)];
